simulink model "A3_A4"  (R2017a)
settings: Solver=VariableStepAuto  StartTime=0.0  StopTime=0.02  MaxStep=1e-4  RelTol=1e-3
libraries: powerlib x11, powerlib_meascontrol x2
settings Model: Creator=Amir Reza  LastModifiedBy=Amir Reza

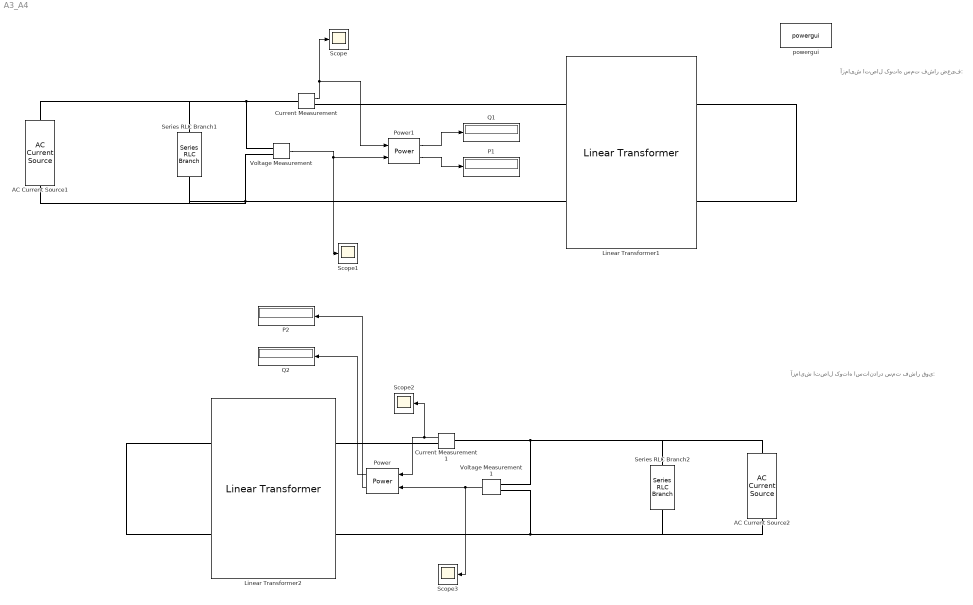
== system A3_A4 ==
  note: آزمایش اتصال کوتاه سمت فشار ضعیف:
  note: آزمایش اتصال کوتاه استاندارد سمت فشار قوی:
  AC Current Source1 : powerlib/Electrical Sources/AC Current Source  Amplitude=312.5  Phase=0  Frequency=50  SampleTime=0  Measurements=None
      settings: SourceProductName=Simscape Power Systems  SourceProductBaseCode=PS
  AC Current Source2 : powerlib/Electrical Sources/AC Current Source  Amplitude=31.25  Phase=0  Frequency=50  SampleTime=0  Measurements=None
      settings: SourceProductName=Simscape Power Systems  SourceProductBaseCode=PS
  Current Measurement : powerlib/Measurements/Current Measurement  PhasorSimulation=off  OutputType=Complex  PSBequivalent=0
  Current Measurement1 : powerlib/Measurements/Current Measurement  PhasorSimulation=off  OutputType=Complex  PSBequivalent=0
  Linear Transformer1 : powerlib/Elements/Linear Transformer  UNITS=SI  NominalPower=[75e3 50 ]  winding1=[240 6e-3 7.57e-5]  winding2=[2400 0.23 9.74e-3]  ThreeWindings=off  winding3=[3.15e+05 1.0502e+06 354.69]  RmLm=[25 3.97e-2]  Measurements=None  DataType=on
  Linear Transformer2 : powerlib/Elements/Linear Transformer  UNITS=SI  NominalPower=[75e3 50 ]  winding1=[240 6e-3 7.57e-5]  winding2=[2400 0.23 9.74e-3]  ThreeWindings=off  winding3=[3.15e+05 1.0502e+06 354.69]  RmLm=[25 3.97e-2]  Measurements=None  DataType=on
  P1 : Display
  "P2 " : Display
  Power : powerlib_meascontrol/Measurements/Power  Freq=50  Vinit=[1, 0]  Iinit=[1, 0]  Ts=0
      settings: SourceProductName=Simscape Power Systems
  Power1 : powerlib_meascontrol/Measurements/Power  Freq=50  Vinit=[1, 0]  Iinit=[1, 0]  Ts=0
      settings: SourceProductName=Simscape Power Systems
  Q1 : Display
  Q2 : Display
  Scope{,1..3} (4 alike) : Scope
  Series RLC Branch1 : powerlib/Elements/Series RLC Branch  LConnTagsString=__new0  RConnTagsString=__new0  BranchType=R  Resistance=1e6  Inductance=1e-3  SetiL0=off  InitialCurrent=0  Capacitance=1e-6  Setx0=off  InitialVoltage=0  Measurements=None
  Series RLC Branch2 : powerlib/Elements/Series RLC Branch  LConnTagsString=__new0  RConnTagsString=__new0  BranchType=R  Resistance=1e6  Inductance=1e-3  SetiL0=off  InitialCurrent=0  Capacitance=1e-6  Setx0=off  InitialVoltage=0  Measurements=None
  Voltage Measurement : powerlib/Measurements/Voltage Measurement  PhasorSimulation=off  OutputType=Complex  PSBequivalent=0
  Voltage Measurement1 : powerlib/Measurements/Voltage Measurement  PhasorSimulation=off  OutputType=Complex  PSBequivalent=0
  powergui : powerlib/powergui  Priority=1  SimulationMode=Continuous  SampleTime=50e-6  frequency=50  Iterations=50  frequencyindice=50  Pbase=100e6  ErrMax=1e-4  UnitsV=kV  UnitsW=MW  buscounter=0  FunctionMessages=off  echomessages=off  EnableUseOfTLC=off  CurrentSourceSwitches=off  DisableSnubberDevices=off  DisableRonSwitches=off  DisableVfSwitches=off  DisplayEquations=off  SolverType=Tustin/Backward Euler (TBE)  Interpol=off  ExternalGateDelay=off  methode=off  Ts=100  x0status=blocks  SPID=on  SwTol=0  HookPort=off  RestoreLinks=warning  ResistiveCurrentMeasurement=off  Frange=[0:50]  Ylog=off  Xlog=off  ShowGrid=off  save=off  variable=ZData  structure=0  ZoomFFT=off  StartTime=0.0  cycles=1  DisplayStyle=1  fundamental=60  FreqAxis=off  MaxFrequency=1000  frequencyindicesteady=50  RmsSteady=1  display=off
  wires:
  Current Measurement/1 -> Power1/2, Scope/1
  Voltage Measurement/1 -> Power1/1, Scope1/1
  Current Measurement1/1 -> Power/2, Scope2/1
  Voltage Measurement1/1 -> Power/1, Scope3/1
  Power/2 -> Q2/1
  Power/1 -> "P2 "/1
  Power1/2 -> Q1/1
  Power1/1 -> P1/1
  connections:
  Voltage Measurement/LConn2 -- Series RLC Branch1/RConn1 -- AC Current Source1/LConn1 -- Linear Transformer1/LConn2
  Voltage Measurement/LConn1 -- Series RLC Branch1/LConn1 -- AC Current Source1/RConn1 -- Current Measurement/LConn1
  Linear Transformer1/LConn1 -- Current Measurement/RConn1
  Voltage Measurement1/LConn1 -- Series RLC Branch2/LConn1 -- AC Current Source2/RConn1 -- Current Measurement1/LConn1
  Linear Transformer2/RConn1 -- Current Measurement1/RConn1
  Linear Transformer2/RConn2 -- Voltage Measurement1/LConn2 -- Series RLC Branch2/RConn1 -- AC Current Source2/LConn1
  Linear Transformer2/LConn1 -- Linear Transformer2/LConn2
  Linear Transformer1/RConn2 -- Linear Transformer1/RConn1
